simulink subsystem "rss_NoLdDia"  (R2023a)
settings: Solver=VariableStepAuto  StartTime=0.0  StopTime=10.0  RelTol=1e-3
undefined symbols (not defined in the file): Cdbl_iPhCurrMaxVal, Cdbl_nElecAgSpdMaxVal, ENM_TYPE_FALT, Gs16_iNoLdPhCurr_CUR, Gs16_iNoLdPhCurr_CUR_nActElecSpd_X, Gs16_nNoLdJudgActElecSpd_C, Gu16_ctNoLdConfCnt_C, Gu16_ctNoLdRcvyCnt_C
libraries: lib_debounce x1, lib_fault_definiteness x1
settings Model: Creator=xiaoqiang.yuan  LastModifiedBy=xiaoqiang.yuan

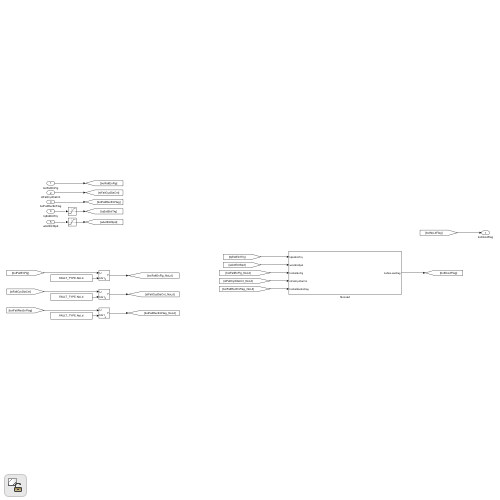
[thumbnail: Simulink's stored preview of the top-level diagram]
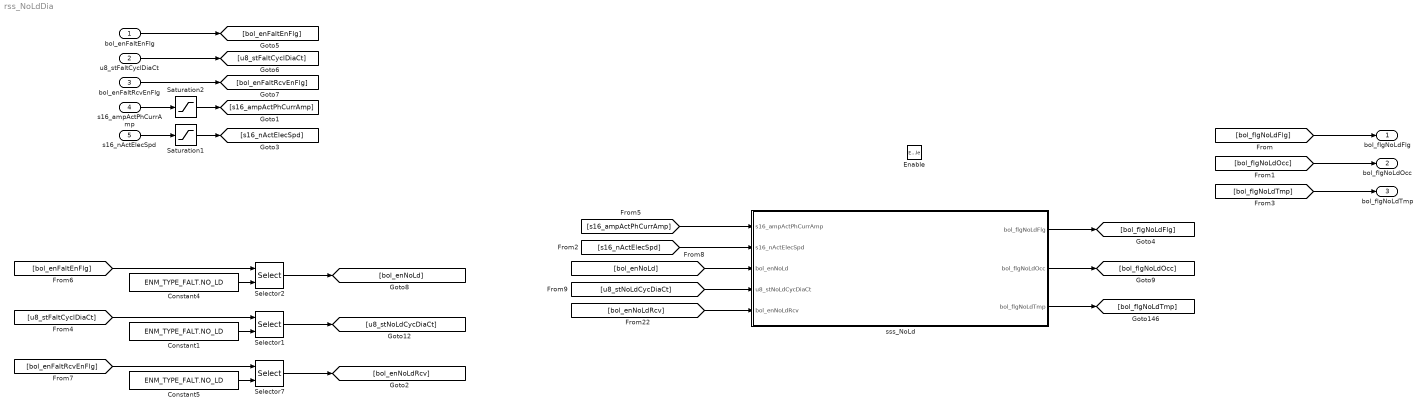
== system rss_NoLdDia ==
  bol_enFaltEnFlg : Inport  OutDataTypeStr=boolean
  u8_stFaltCyclDiaCt : Inport  Port=2  OutDataTypeStr=uint8
  bol_enFaltRcvEnFlg : Inport  Port=3  OutDataTypeStr=boolean
  s16_ampActPhCurrAmp : Inport  Port=4  OutDataTypeStr=dt_Standardize_s16p15b0
  s16_nActElecSpd : Inport  Port=5  OutDataTypeStr=dt_Standardize_s16p15b0
  Enable : EnablePort
  Constant1 : Constant  Value=ENM_TYPE_FALT.NO_LD
  Constant4 : Constant  Value=ENM_TYPE_FALT.NO_LD
  Constant5 : Constant  Value=ENM_TYPE_FALT.NO_LD
  Saturation1 : Saturate  UpperLimit=Cdbl_nElecAgSpdMaxVal  LowerLimit=-Cdbl_nElecAgSpdMaxVal
  Saturation2 : Saturate  UpperLimit=Cdbl_iPhCurrMaxVal  LowerLimit=0
  Selector1 : Selector  IndexMode=Zero-based  InputPortWidth=Cdbl_numFaltDiaNum  IndexOptions=Index vector (port)  Indices=[1 3]  OutputSizes=1
  Selector2 : Selector  IndexMode=Zero-based  InputPortWidth=Cdbl_numFaltDiaNum  IndexOptions=Index vector (port)  Indices=[1 3]  OutputSizes=1
  Selector7 : Selector  IndexMode=Zero-based  InputPortWidth=Cdbl_numFaltDiaNum  IndexOptions=Index vector (port)  Indices=[1 3]  OutputSizes=1
  sss_NoLd : Subsystem
  bol_flgNoLdFlg : Outport  OutDataTypeStr=boolean
  bol_flgNoLdOcc : Outport  Port=2  OutDataTypeStr=boolean
  bol_flgNoLdTmp : Outport  Port=3  OutDataTypeStr=boolean
  wires:
  [bol_flgNoLdFlg] -> bol_flgNoLdFlg/1
  s16_nActElecSpd/1 -> Saturation1/1
  s16_ampActPhCurrAmp/1 -> Saturation2/1
  Selector7/1 -> [bol_enNoLdRcv]
  Constant1/1 -> Selector1/2
  Constant4/1 -> Selector2/2
  Constant5/1 -> Selector7/2
  [bol_enFaltEnFlg] -> Selector2/1
  Selector1/1 -> [u8_stNoLdCycDiaCt]
  [bol_enNoLd] -> sss_NoLd/3(bol_enNoLd)
  [u8_stFaltCyclDiaCt] -> Selector1/1
  [u8_stNoLdCycDiaCt] -> sss_NoLd/4(u8_stNoLdCycDiaCt)
  [bol_enFaltRcvEnFlg] -> Selector7/1
  Selector2/1 -> [bol_enNoLd]
  [bol_enNoLdRcv] -> sss_NoLd/5(bol_enNoLdRcv)
  sss_NoLd/1(bol_flgNoLdFlg) -> [bol_flgNoLdFlg]
  [s16_ampActPhCurrAmp] -> sss_NoLd/1(s16_ampActPhCurrAmp)
  [s16_nActElecSpd] -> sss_NoLd/2(s16_nActElecSpd)
  bol_enFaltRcvEnFlg/1 -> [bol_enFaltRcvEnFlg]
  u8_stFaltCyclDiaCt/1 -> [u8_stFaltCyclDiaCt]
  bol_enFaltEnFlg/1 -> [bol_enFaltEnFlg]
  Saturation1/1 -> [s16_nActElecSpd]
  Saturation2/1 -> [s16_ampActPhCurrAmp]
  sss_NoLd/2(bol_flgNoLdOcc) -> [bol_flgNoLdOcc]
  [bol_flgNoLdOcc] -> bol_flgNoLdOcc/1
  [bol_flgNoLdTmp] -> bol_flgNoLdTmp/1
  sss_NoLd/3(bol_flgNoLdTmp) -> [bol_flgNoLdTmp]

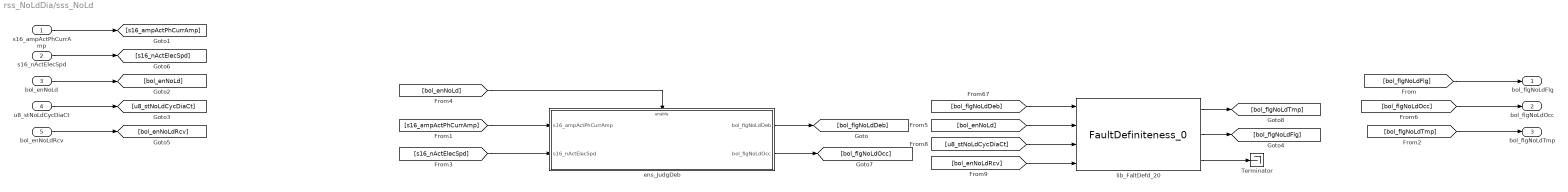
== system rss_NoLdDia/sss_NoLd ==
  s16_ampActPhCurrAmp : Inport
  s16_nActElecSpd : Inport  Port=2
  bol_enNoLd : Inport  Port=3
  u8_stNoLdCycDiaCt : Inport  Port=4
  bol_enNoLdRcv : Inport  Port=5
  Terminator : Terminator
  ens_JudgDeb : Subsystem
  lib_FaltDefd_20 : lib_fault_definiteness/FaultDefiniteness_0  lb_FaltWaitRecvCnt=Gu16_ctNoLdConfCnt_C
  bol_flgNoLdFlg : Outport
  bol_flgNoLdOcc : Outport  Port=2
  bol_flgNoLdTmp : Outport  Port=3
  wires:
  [bol_flgNoLdTmp] -> bol_flgNoLdTmp/1
  [bol_flgNoLdOcc] -> bol_flgNoLdOcc/1
  ens_JudgDeb/2(bol_flgNoLdOcc) -> [bol_flgNoLdOcc]
  lib_FaltDefd_20/1 -> [bol_flgNoLdTmp]
  lib_FaltDefd_20/2 -> [bol_flgNoLdFlg]
  lib_FaltDefd_20/3 -> Terminator/1
  [bol_enNoLd] -> ens_JudgDeb/Enable
  [s16_nActElecSpd] -> ens_JudgDeb/2(s16_nActElecSpd)
  s16_nActElecSpd/1 -> [s16_nActElecSpd]
  [s16_ampActPhCurrAmp] -> ens_JudgDeb/1(s16_ampActPhCurrAmp)
  ens_JudgDeb/1(bol_flgNoLdDeb) -> [bol_flgNoLdDeb]
  bol_enNoLdRcv/1 -> [bol_enNoLdRcv]
  u8_stNoLdCycDiaCt/1 -> [u8_stNoLdCycDiaCt]
  bol_enNoLd/1 -> [bol_enNoLd]
  [bol_flgNoLdFlg] -> bol_flgNoLdFlg/1
  s16_ampActPhCurrAmp/1 -> [s16_ampActPhCurrAmp]
  [bol_enNoLdRcv] -> lib_FaltDefd_20/4
  [u8_stNoLdCycDiaCt] -> lib_FaltDefd_20/3
  [bol_enNoLd] -> lib_FaltDefd_20/2
  [bol_flgNoLdDeb] -> lib_FaltDefd_20/1

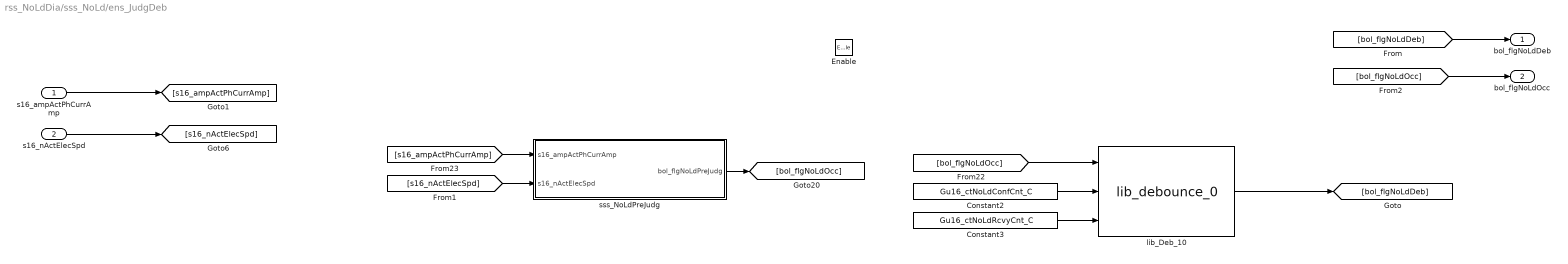
== system rss_NoLdDia/sss_NoLd/ens_JudgDeb ==
  s16_ampActPhCurrAmp : Inport
  s16_nActElecSpd : Inport  Port=2
  Enable : EnablePort
  Constant2 : Constant  Value=Gu16_ctNoLdConfCnt_C
  Constant3 : Constant  Value=Gu16_ctNoLdRcvyCnt_C
  lib_Deb_10 : lib_debounce/lib_debounce_0
  sss_NoLdPreJudg : Subsystem
  bol_flgNoLdDeb : Outport
  bol_flgNoLdOcc : Outport  Port=2
  wires:
  [bol_flgNoLdOcc] -> bol_flgNoLdOcc/1
  [s16_nActElecSpd] -> sss_NoLdPreJudg/2(s16_nActElecSpd)
  s16_nActElecSpd/1 -> [s16_nActElecSpd]
  [s16_ampActPhCurrAmp] -> sss_NoLdPreJudg/1(s16_ampActPhCurrAmp)
  s16_ampActPhCurrAmp/1 -> [s16_ampActPhCurrAmp]
  [bol_flgNoLdDeb] -> bol_flgNoLdDeb/1
  sss_NoLdPreJudg/1(bol_flgNoLdPreJudg) -> [bol_flgNoLdOcc]
  Constant3/1 -> lib_Deb_10/3
  [bol_flgNoLdOcc] -> lib_Deb_10/1
  lib_Deb_10/1 -> [bol_flgNoLdDeb]
  Constant2/1 -> lib_Deb_10/2

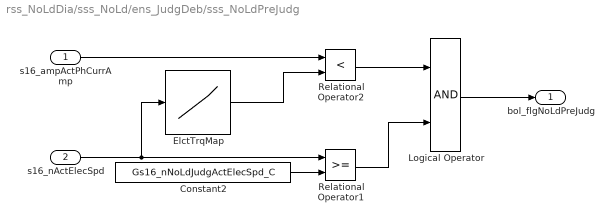
== system rss_NoLdDia/sss_NoLd/ens_JudgDeb/sss_NoLdPreJudg ==
  s16_ampActPhCurrAmp : Inport
  s16_nActElecSpd : Inport  Port=2
  Constant2 : Constant  Value=Gs16_nNoLdJudgActElecSpd_C
  ElctTrqMap : Lookup_n-D  NumberOfTableDimensions=1  BreakpointsForDimension1=Gs16_iNoLdPhCurr_CUR_nActElecSpd_X  BreakpointsForDimension1DataTypeStr=Inherit: Inherit from 'Breakpoint data'  Table=Gs16_iNoLdPhCurr_CUR  TableDataTypeStr=Inherit: Inherit from 'Table data'  ExtrapMethod=Clip  UseLastTableValue=on  OutDataTypeStr=Inherit: Inherit from 'Table data'  RndMeth=Simplest  SaturateOnIntegerOverflow=on  InputSameDT=off
  Logical Operator : Logic  AllPortsSameDT=off  OutDataTypeStr=boolean
  Relational Operator1 : RelationalOperator  OutDataTypeStr=boolean  RndMeth=Simplest  InputSameDT=off
  Relational Operator2 : RelationalOperator  Operator=<  OutDataTypeStr=boolean  RndMeth=Simplest  InputSameDT=off
  bol_flgNoLdPreJudg : Outport
  wires:
  ElctTrqMap/1 -> Relational Operator2/2
  Logical Operator/1 -> bol_flgNoLdPreJudg/1
  Relational Operator1/1 -> Logical Operator/2
  Relational Operator2/1 -> Logical Operator/1
  Constant2/1 -> Relational Operator1/2
  s16_nActElecSpd/1 -> Relational Operator1/1, ElctTrqMap/1
  s16_ampActPhCurrAmp/1 -> Relational Operator2/1
